simulink model "stateflow_ex3"  (R2022a)
settings: Solver=VariableStepAuto  StartTime=0.0  StopTime=10.0  RelTol=1e-3
settings Model: Creator=ArriGE66  LastModifiedBy=ArriGE66

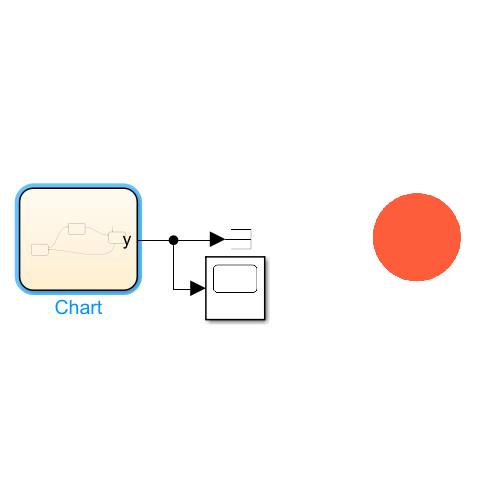
[thumbnail: Simulink's stored preview of the top-level diagram]
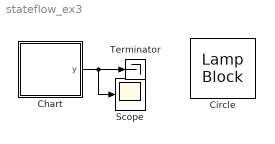
== system stateflow_ex3 ==
  Chart : Stateflow chart  TreatAsAtomicUnit=on
  Circle : LampBlock  LabelPosition=Hide  Icon=Circle
  Scope : Scope
  Terminator : Terminator
  wires:
  Chart/1(y) -> Scope/1, Terminator/1

== stateflow chart stateflow_ex3/Chart ==
  state yellow
    y=2;
  state red
    y=3;
  state green
    y=1;
  (default) -> red
  green -> yellow : [after(3,sec)]
  yellow -> red : [after(1,sec)]
  red -> green : [after(5,sec)]
  data: y output
